simulink model "Inclusao_Sensores"  (R2020a)
settings: Solver=VariableStepAuto  StartTime=0.0  StopTime=200  RelTol=1e-3
values from neighbouring files (symbols this model uses):
  A = [Ybb  Yp+W0/U0      Yr-1  (g*cos(tt0))/U0 ... (first row only)    [Aterragem_sematuadores.m]    (also in EKC39.m)
  act_t = 0.1    [dados_sensores.m]
  act_vmax = 1    [dados_sensores.m]
  B = [YdA      YdR ... (first row only)    [Aterragem_sematuadores.m]    (also in EKC39.m)
  bb0 = 0    [Aterragem_sematuadores.m]    (also in EKC39.m)
  C = eye(4)    [Aterragem_sematuadores.m]    (also in EKC39.m)
  D = zeros(4,2)    [Aterragem_sematuadores.m]    (also in EKC39.m)
  dda_max = 20 * deg    (= 0.349065850399)    [Aterragem_sematuadores.m]    (also in EKC39.m)
  ddr_max = 20 * deg    (= 0.349065850399)    [Aterragem_sematuadores.m]    (also in EKC39.m)
  f = 40    [dados_sensores.m]
  k_integrativo = k_lqr(:,5:6)    [EKC39.m]
  k_interior4 = k_lqr(:,2:3)    [EKC39.m]
  k_proporcional = [k_lqr(:,1) k_lqr(:,4)]    [EKC39.m]
  p0 = 0    [Aterragem_sematuadores.m]    (also in EKC39.m)
  phi0 = 0    [Aterragem_sematuadores.m]    (also in EKC39.m)
  r0 = 0    [Aterragem_sematuadores.m]    (also in EKC39.m)
  s1_k = (s1_outmax-s1_outmin)/(s1_inmax-s1_inmin)    (= 5.72957795131)    [dados_sensores.m]
  s1_offset = s1_outmax-s1_k*s1_inmax    (= 2.5)    [dados_sensores.m]
  s1_outmax = 5    [dados_sensores.m]
  s1_outmin = 0    [dados_sensores.m]
  s1_t_const = 0.01    [dados_sensores.m]
  s2_k = (s2_outmax-s2_outmin)/(s2_inmax-s2_inmin)    (= 3.43774677078)    [dados_sensores.m]
  s2_offset = s2_outmax-s2_k*s2_inmax    (= 0)    [dados_sensores.m]
  s2_outmax = 3    [dados_sensores.m]
  s2_outmin = -3    [dados_sensores.m]
  s3_k = (s3_outmax-s3_outmin)/(s3_inmax-s3_inmin)    (= 8.91267681315)    [dados_sensores.m]
  s3_offset = s3_outmax-s3_k*s3_inmax    (= 14)    [dados_sensores.m]
  s3_outmax = 28    [dados_sensores.m]
  s3_outmin = 0    [dados_sensores.m]
libraries: simulink x3
settings Model: Creator=vicen  LastModifiedBy=vicen

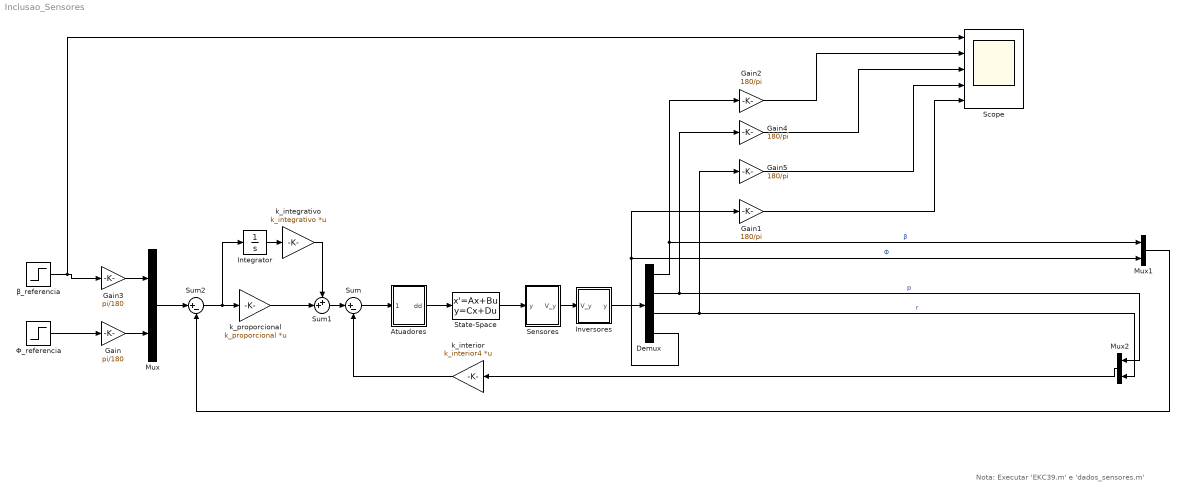
== system Inclusao_Sensores ==
  note: Nota: Executar 'EKC39.m' e 'dados_sensores.m'
  Atuadores : Subsystem
  Demux : Demux
  Gain : Gain  Gain=pi/180
  Gain{1..2,4..5} (4 alike) : Gain  Gain=180/pi
  Gain3 : Gain  Gain=pi/180
  Integrator : Integrator
  Inversores : Subsystem
  Mux : Mux  Inputs=2
  Mux1 : Mux  Inputs=2
  Mux2 : Mux  Inputs=2
  Scope : Scope  NumInputPorts=5
  Sensores : Subsystem
  State-Space : StateSpace  A=A  B=B  C=C  D=D  InitialCondition=0
  Sum : Sum  Inputs=|+-
  Sum1 : Sum  Inputs=++|
  Sum2 : Sum  Inputs=|+-
  k_integrativo : Gain  Gain=k_integrativo  Multiplication=Matrix(K*u)
  k_interior : Gain  Gain=k_interior4  Multiplication=Matrix(K*u)
  k_proporcional : Gain  Gain=k_proporcional  Multiplication=Matrix(K*u)
  Φ_referencia : Step  Time=100  After=0  SampleTime=0
  β_referencia : Step  After=10  SampleTime=0
  wires:
  k_interior/1 -> Sum/2
  β_referencia/1 -> Scope/1, Gain3/1
  k_integrativo/1 -> Sum1/1
  Integrator/1 -> k_integrativo/1
  k_proporcional/1 -> Sum1/2
  Sum2/1 -> Integrator/1, k_proporcional/1
  Mux/1 -> Sum2/1
  Φ_referencia/1 -> Gain/1
  Demux/1 -> Gain2/1, Mux1/1  "β"
  Demux/2 -> Gain4/1, Mux2/1  "p"
  Demux/3 -> Gain5/1, Mux2/2  "r"
  Mux2/1 -> k_interior/1
  Demux/4 -> Gain1/1, Mux1/2  "Φ"
  Mux1/1 -> Sum2/2
  Sum1/1 -> Sum/1
  Gain3/1 -> Mux/1
  Gain/1 -> Mux/2
  State-Space/1 -> Sensores/1(y)
  Sum/1 -> Atuadores/1(V_dd)
  Sensores/1(V_y) -> Inversores/1(V_y)
  Inversores/1(y) -> Demux/1
  Gain2/1 -> Scope/2
  Gain4/1 -> Scope/3
  Gain5/1 -> Scope/4
  Gain1/1 -> Scope/5
  Atuadores/1(dd) -> State-Space/1

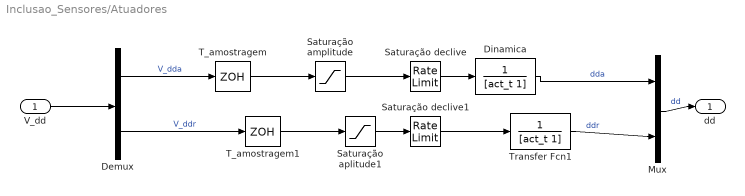
== system Inclusao_Sensores/Atuadores ==
  V_dd : Inport
  Demux : Demux  Outputs=2
  Dinamica : TransferFcn  Denominator=[act_t 1]
  Mux : Mux  Inputs=2
  Saturação amplitude : Saturate  UpperLimit=dda_max  LowerLimit=-dda_max
  Saturação aplitude1 : Saturate  UpperLimit=ddr_max  LowerLimit=-ddr_max
  Saturação declive : RateLimiter  RisingSlewLimit=act_vmax  FallingSlewLimit=-act_vmax  SampleTimeMode=inherited
  Saturação declive1 : RateLimiter  RisingSlewLimit=act_vmax  FallingSlewLimit=-act_vmax  SampleTimeMode=inherited
  T_amostragem : ZeroOrderHold  SampleTime=1/f
  T_amostragem1 : ZeroOrderHold  SampleTime=1/f
  Transfer Fcn1 : TransferFcn  Denominator=[act_t 1]
  dd : Outport
  wires:
  Transfer Fcn1/1 -> Mux/2  "ddr"
  Mux/1 -> dd/1  "dd"
  V_dd/1 -> Demux/1
  Demux/1 -> T_amostragem/1  "V_dda"
  T_amostragem/1 -> Saturação amplitude/1
  T_amostragem1/1 -> Saturação aplitude1/1
  Dinamica/1 -> Mux/1  "dda"
  Saturação amplitude/1 -> Saturação declive/1
  Saturação aplitude1/1 -> Saturação declive1/1
  Saturação declive/1 -> Dinamica/1
  Saturação declive1/1 -> Transfer Fcn1/1
  Demux/2 -> T_amostragem1/1  "V_ddr"

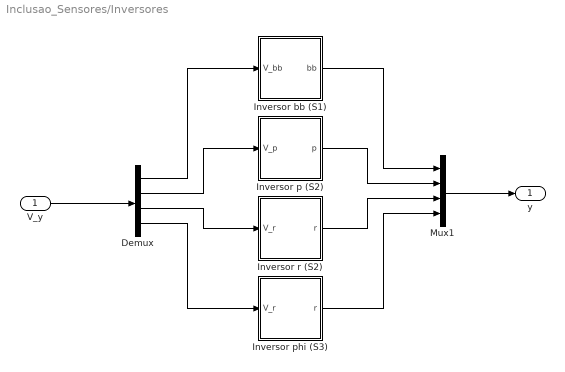
== system Inclusao_Sensores/Inversores ==
  V_y : Inport
  Demux : Demux
  Inversor bb (S1) : Subsystem
  Inversor p (S2) : Subsystem
  Inversor phi (S3) : Subsystem
  Inversor r (S2) : Subsystem
  Mux1 : Mux
  y : Outport
  wires:
  V_y/1 -> Demux/1
  Demux/2 -> Inversor p (S2)/1(V_p)
  Demux/4 -> Inversor phi (S3)/1(V_r)
  Demux/1 -> Inversor bb (S1)/1(V_bb)
  Inversor p (S2)/1(p) -> Mux1/2
  Inversor bb (S1)/1(bb) -> Mux1/1
  Mux1/1 -> y/1
  Inversor r (S2)/1(r) -> Mux1/3
  Demux/3 -> Inversor r (S2)/1(V_r)
  Inversor phi (S3)/1(r) -> Mux1/4

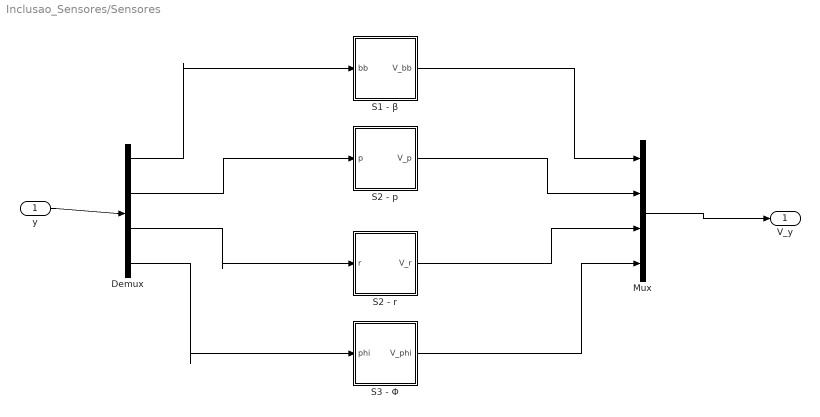
== system Inclusao_Sensores/Sensores ==
  y : Inport
  Demux : Demux
  Mux : Mux
  "S1 - β " : Subsystem
  S2 - p : Subsystem
  S2 - r : Subsystem
  S3 - Φ : Subsystem
  V_y : Outport
  wires:
  Mux/1 -> V_y/1
  "S1 - β "/1(V_bb) -> Mux/1
  S3 - Φ/1(V_phi) -> Mux/4
  S2 - p/1(V_p) -> Mux/2
  S2 - r/1(V_r) -> Mux/3
  y/1 -> Demux/1
  Demux/2 -> S2 - p/1(p)
  Demux/3 -> S2 - r/1(r)
  Demux/1 -> "S1 - β "/1(bb)
  Demux/4 -> S3 - Φ/1(phi)

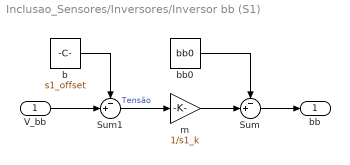
== system Inclusao_Sensores/Inversores/Inversor bb (S1) ==
  V_bb : Inport
  Sum : Sum  Inputs=-+|
  Sum1 : Sum  Inputs=-+|
  b : Constant  Value=s1_offset
  bb0 : Constant  Value=bb0
  m : Gain  Gain=1/s1_k
  bb : Outport
  wires:
  bb0/1 -> Sum/1
  b/1 -> Sum1/1
  V_bb/1 -> Sum1/2
  Sum1/1 -> m/1  "Tensão"
  m/1 -> Sum/2
  Sum/1 -> bb/1

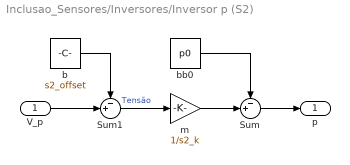
== system Inclusao_Sensores/Inversores/Inversor p (S2) ==
  V_p : Inport
  Sum : Sum  Inputs=-+|
  Sum1 : Sum  Inputs=-+|
  b : Constant  Value=s2_offset
  bb0 : Constant  Value=p0
  m : Gain  Gain=1/s2_k
  p : Outport
  wires:
  bb0/1 -> Sum/1
  b/1 -> Sum1/1
  V_p/1 -> Sum1/2
  Sum1/1 -> m/1  "Tensão"
  m/1 -> Sum/2
  Sum/1 -> p/1

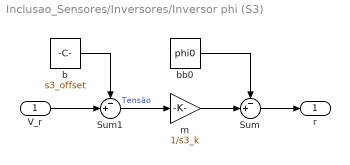
== system Inclusao_Sensores/Inversores/Inversor phi (S3) ==
  V_r : Inport
  Sum : Sum  Inputs=-+|
  Sum1 : Sum  Inputs=-+|
  b : Constant  Value=s3_offset
  bb0 : Constant  Value=phi0
  m : Gain  Gain=1/s3_k
  r : Outport
  wires:
  bb0/1 -> Sum/1
  b/1 -> Sum1/1
  V_r/1 -> Sum1/2
  Sum1/1 -> m/1  "Tensão"
  m/1 -> Sum/2
  Sum/1 -> r/1

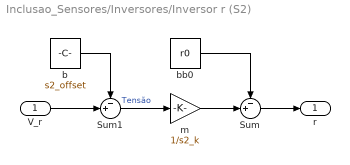
== system Inclusao_Sensores/Inversores/Inversor r (S2) ==
  V_r : Inport
  Sum : Sum  Inputs=-+|
  Sum1 : Sum  Inputs=-+|
  b : Constant  Value=s2_offset
  bb0 : Constant  Value=r0
  m : Gain  Gain=1/s2_k
  r : Outport
  wires:
  bb0/1 -> Sum/1
  b/1 -> Sum1/1
  V_r/1 -> Sum1/2
  Sum1/1 -> m/1  "Tensão"
  m/1 -> Sum/2
  Sum/1 -> r/1

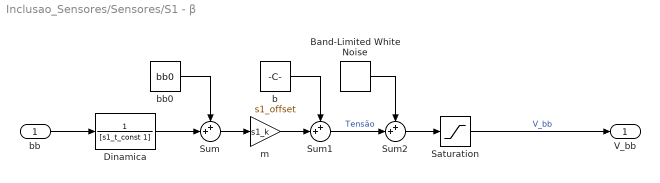
== system Inclusao_Sensores/Sensores/S1 - β  ==
  bb : Inport
  " Dinamica" : TransferFcn  Denominator=[s1_t_const 1]
  Band-Limited White Noise : simulink/Sources/Band-Limited White Noise  Cov=s1_power  Ts=1/f  seed=[23341]
  Saturation : Saturate  UpperLimit=s1_outmax  LowerLimit=s1_outmin
  Sum : Sum  Inputs=++|
  Sum1 : Sum  Inputs=++|
  Sum2 : Sum  Inputs=++|
  b : Constant  Value=s1_offset
  bb0 : Constant  Value=bb0
  m : Gain  Gain=s1_k
  V_bb : Outport
  wires:
  Sum2/1 -> Saturation/1
  bb/1 -> " Dinamica"/1
  bb0/1 -> Sum/1
  Sum/1 -> m/1
  Sum1/1 -> Sum2/2  "Tensão"
  m/1 -> Sum1/2
  b/1 -> Sum1/1
  Band-Limited White Noise/1 -> Sum2/1
  " Dinamica"/1 -> Sum/2
  Saturation/1 -> V_bb/1  "V_bb"

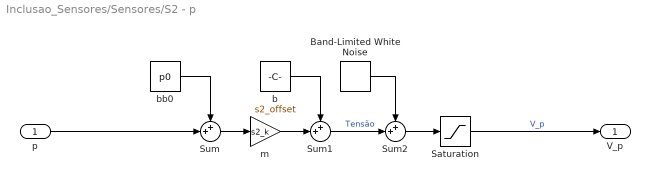
== system Inclusao_Sensores/Sensores/S2 - p ==
  p : Inport
  Band-Limited White Noise : simulink/Sources/Band-Limited White Noise  Cov=s2_power  Ts=1/f  seed=[01933]
  Saturation : Saturate  UpperLimit=s2_outmax  LowerLimit=s2_outmin
  Sum : Sum  Inputs=++|
  Sum1 : Sum  Inputs=++|
  Sum2 : Sum  Inputs=++|
  b : Constant  Value=s2_offset
  bb0 : Constant  Value=p0
  m : Gain  Gain=s2_k
  V_p : Outport
  wires:
  Sum2/1 -> Saturation/1
  bb0/1 -> Sum/1
  Sum/1 -> m/1
  Sum1/1 -> Sum2/2  "Tensão"
  m/1 -> Sum1/2
  b/1 -> Sum1/1
  Band-Limited White Noise/1 -> Sum2/1
  p/1 -> Sum/2
  Saturation/1 -> V_p/1  "V_p"

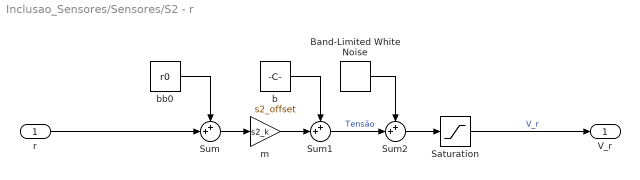
== system Inclusao_Sensores/Sensores/S2 - r ==
  r : Inport
  Band-Limited White Noise : simulink/Sources/Band-Limited White Noise  Cov=s2_power  Ts=1/f  seed=[26007]
  Saturation : Saturate  UpperLimit=s2_outmax  LowerLimit=s2_outmin
  Sum : Sum  Inputs=++|
  Sum1 : Sum  Inputs=++|
  Sum2 : Sum  Inputs=++|
  b : Constant  Value=s2_offset
  bb0 : Constant  Value=r0
  m : Gain  Gain=s2_k
  V_r : Outport
  wires:
  Sum2/1 -> Saturation/1
  bb0/1 -> Sum/1
  Sum/1 -> m/1
  Sum1/1 -> Sum2/2  "Tensão"
  m/1 -> Sum1/2
  b/1 -> Sum1/1
  Band-Limited White Noise/1 -> Sum2/1
  r/1 -> Sum/2
  Saturation/1 -> V_r/1  "V_r"

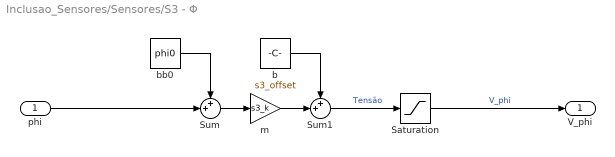
== system Inclusao_Sensores/Sensores/S3 - Φ ==
  phi : Inport
  Saturation : Saturate  UpperLimit=s3_outmax  LowerLimit=s3_outmin
  Sum : Sum  Inputs=++|
  Sum1 : Sum  Inputs=++|
  b : Constant  Value=s3_offset
  bb0 : Constant  Value=phi0
  m : Gain  Gain=s3_k
  V_phi : Outport
  wires:
  bb0/1 -> Sum/1
  Sum/1 -> m/1
  Sum1/1 -> Saturation/1  "Tensão"
  m/1 -> Sum1/2
  b/1 -> Sum1/1
  phi/1 -> Sum/2
  Saturation/1 -> V_phi/1  "V_phi"
